simulink model "ME226Sim"  (R2023b)
settings: Solver=FixedStepAuto  StartTime=0.0  StopTime=10  FixedStep=0.00001  RelTol=1e-3
values from neighbouring files (symbols this model uses):
  A = [0 0 0 0 1 0 0 0 ... (first row only)    [ME226_Problem6.m]
  B = [ ... (first row only)    [ME226_Problem6.m]
  C = [cs -cs ... (first row only)    [Final_Q3.m]    (also in ME226_Problem6.m = [1 0 0 0 0 0 0 0)
  D = zeros(8,2)    [ME226_Problem6.m]
settings Model: Creator=elija  LastModifiedBy=elija

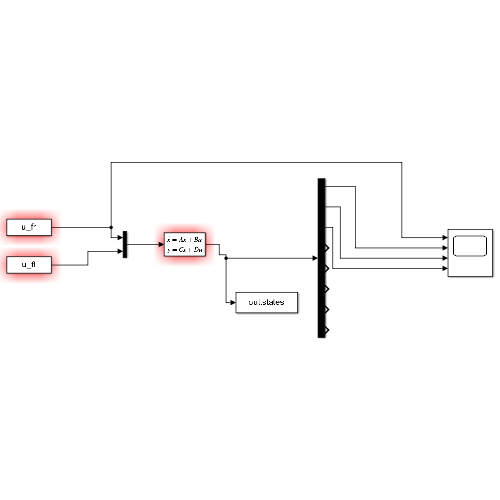
[thumbnail: Simulink's stored preview of the top-level diagram]
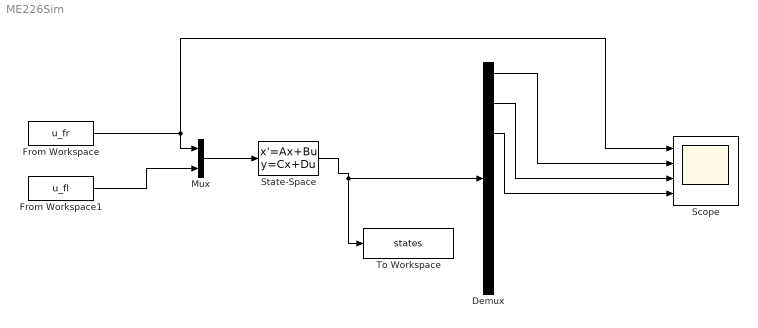
== system ME226Sim ==
  Demux : Demux  Outputs=8
  From Workspace : FromWorkspace  VariableName=u_fr
  From Workspace1 : FromWorkspace  VariableName=u_fl
  Mux : Mux  Inputs=2
  Scope : Scope  NumInputPorts=4
  State-Space : StateSpace  A=A  B=B  C=C  D=D  InitialCondition=0
  To Workspace : ToWorkspace  VariableName=states  SaveFormat=Timeseries  SampleTime=-1
  wires:
  State-Space/1 -> To Workspace/1, Demux/1
  Mux/1 -> State-Space/1
  From Workspace/1 -> Scope/1, Mux/1
  From Workspace1/1 -> Mux/2
  Demux/1 -> Scope/2
  Demux/2 -> Scope/3
  Demux/3 -> Scope/4
